simulink library "Roll_Resistance"  (R2018b)
settings: Solver=VariableStepAuto  StartTime=0.0  StopTime=10.0  RelTol=1e-3
settings Model: Creator=Alexander Koch  LastModifiedBy=ga69qig
settings SFSimCC: SimUseLocalCustomCode=off
settings RTWCC: RTWUseLocalCustomCode=off
settings CodeAppCC: StateflowObjectComments=on

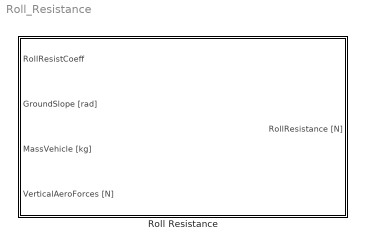
== system Roll_Resistance ==
  Roll Resistance : Subsystem  mask(SB){Gravity=9.81, LocalSampleTime=-1}
      mask prompts: Gravity "Gravity [N/kg]"; LocalSampleTime "Local System Sample-Time [s]"
      mask help:
      | <Author> Alexander Koch, Benedikt Danquah based on Stefan Müller [1], Stephan Rohr [2]  </Author>
      | <Date> 21/03/2017 </Date>
      | <Sources>
      | [1] S. Mueller, S. Rohr, und et al, Hrsg, Analysing the Influence of Driver Behaviour and Tuning Measures on Battery Aging and Residual Value of Electric Vehicles, 2017
      | </Sources>
      |
      | <Description>
      | Requires roll resistance coefficient, ground slope, mass of vehicle, vertical aero forces and gravity and calculates the roll resistance. Vertical aero forces describe the result of lift and down force due to wings etc.
      | </Description>
      mask init:
      | GlobalSampleTime = CalcGlobalSampleTime(LocalSampleTime);
      mask Help:
      | <Parameters>
      | Gravity [N/kg]
      | Local System Sample-Time [s]
      | 	<Min> GlobalSampleTime </Min>
      | Global Sample-Time [s]
      | </Parameters>
      | 
      | <Inputs>
      | RollResistCoeff [-]
      | GroundSlope [rad]
      | 	<sign orientation> [+] uphill </sign orientation>
      | MassVehicle [kg]
      | VerticalAeroForces [N]
      | 	<sign orientation> [+] lift </sign orientation>
      | </Inputs>
      | 
      | <Outputs>
      | RollResistance [N]
      | </Outputs>
      | <Sources>
      | [1] S. Mueller, S. Rohr, W. Schmid, and M. Lienkamp, “Analysing the Influence of Driver Behaviour and Tuning Measures on Battery Aging and Residual Value of Electric Vehicles,” in Proc. EVS30 Symposium, Stuttgart, 2017, pp. 1–12.
      | [2] S. Rohr, “Technisch-wirtschaftliche Analyse des Zweitnutzungs- potentials von Lithium-Ionen-Traktionsbatterien,” Dissertation, Institute of Automotive Technology, Technical University Munich, Munich, 2018.
      | </Sources>
      mask TypeOptions Gravity: Gravity/Gain
      mask TypeOptions LocalSampleTime: RollResistCoeff/SampleTime | GroundSlope [rad]/SampleTime | MassVehicle [kg]/SampleTime | VerticalAeroForces [N]/SampleTime
      mask DialogControl Container4 Prompt: Documentation:
      mask DialogControl Control2 Prompt: %<MaskHelp>
      mask DialogControl Container5 Prompt: Sample Time
      mask Display:
      | [picturexpos,pictureypos,picturewidth,pictureheight] = ...
      |     CalcBlockPicturePosition(gcb,1,0.01,0.1,90,80); % calculating picture position depending on Block size and minimum margin size
      | image('Roll_Resistance.svg',[picturexpos pictureypos picturewidth pictureheight]); % plot picture to block

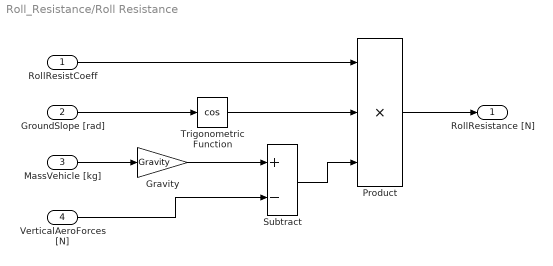
== system Roll_Resistance/Roll Resistance ==
  RollResistCoeff : Inport  SampleTime=LocalSampleTime
  GroundSlope [rad] : Inport  Port=2  SampleTime=LocalSampleTime
  MassVehicle [kg] : Inport  Port=3  SampleTime=LocalSampleTime
  VerticalAeroForces [N] : Inport  Port=4  SampleTime=LocalSampleTime
  Gravity : Gain  Gain=Gravity
  Product : Product  Inputs=3
  Subtract : Sum  Inputs=+-
  Trigonometric Function : Trigonometry  Operator=cos
  RollResistance [N] : Outport  SampleTime=GlobalSampleTime
  wires:
  RollResistCoeff/1 -> Product/1
  MassVehicle [kg]/1 -> Gravity/1
  Subtract/1 -> Product/3
  Trigonometric Function/1 -> Product/2
  Gravity/1 -> Subtract/1
  Product/1 -> RollResistance [N]/1
  GroundSlope [rad]/1 -> Trigonometric Function/1
  VerticalAeroForces [N]/1 -> Subtract/2
